simulink model "quartercar_active"  (Simulink 8.1)
settings: Solver=ode45  StartTime=0.0  StopTime=100  RelTol=1e-3
InitFcn:
  | mb=2500;
  | mw=320;
  | k1=80000;
  | k2=500000;
  | b1=320;
  | b2=15020;
  | h=1;
  | n=100;
  | g=5.01;
  | ksw=100.65;
settings Model: Creator=Sukriti Singh  LastModifiedBy=Sukriti Singh
settings DataIOCC: SignalLoggingSaveFormat=Dataset  InspectSignalLogs=on
settings OptimizationCC: ExpressionDepthLimit=128
settings DebuggingCC: FcnCallInpInsideContextMsg=EnableAllAsError
settings GRTTargetCC: CombineOutputUpdateFcns=on  GRTInterface=off

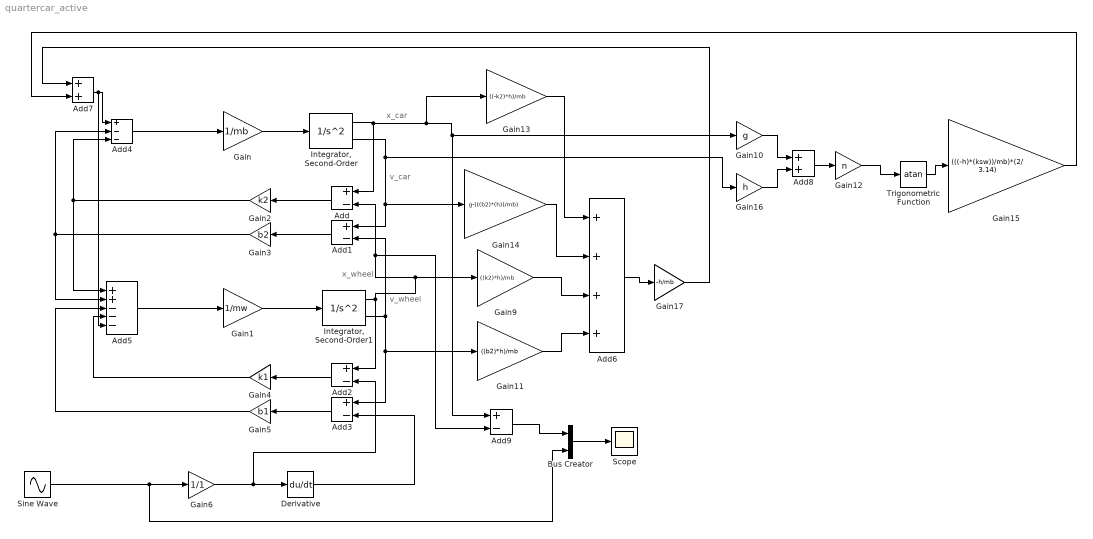
== system quartercar_active ==
  note: v_wheel
  note: x_wheel
  note: x_car
  note: v_car
  Add{,1..3,9} (5 alike) : Sum  Inputs=+-
  Add4 : Sum  Inputs=+--
  Add5 : Sum  Inputs=++---
  Add6 : Sum  Inputs=++++
  Add7 : Sum
  Add8 : Sum
  Bus Creator : BusCreator  Inputs=2
  Derivative : Derivative
  Gain : Gain  Gain=1/mb
  Gain1 : Gain  Gain=1/mw
  Gain10 : Gain  Gain=g
  Gain11 : Gain  Gain=((b2)*h)/mb
  Gain12 : Gain  Gain=n
  Gain13 : Gain  Gain=((-k2)*h)/mb
  Gain14 : Gain  Gain=g-(((b2)*(h))/mb)
  Gain15 : Gain  Gain=(((-h)*(ksw))/mb)*(2/ 3.14)
  Gain16 : Gain  Gain=h
  Gain17 : Gain  Gain=-h/mb
  Gain2 : Gain  Gain=k2
  Gain3 : Gain  Gain=b2
  Gain4 : Gain  Gain=k1
  Gain5 : Gain  Gain=b1
  Gain6 : Gain  Gain=1/1
  Gain9 : Gain  Gain=((k2)*h)/mb
  "Integrator, Second-Order" : SecondOrderIntegrator
  "Integrator, Second-Order1" : SecondOrderIntegrator
  Scope : Scope
      settings: YMax=4.5
  Sine Wave : Sin  Amplitude=0.01  Frequency=20  SampleTime=0
  Trigonometric Function : Trigonometry  Operator=atan
  wires:
  Derivative/1 -> Add3/2
  Add3/1 -> Gain5/1
  Add2/1 -> Gain4/1
  Gain1/1 -> "Integrator, Second-Order1"/1
  Add1/1 -> Gain3/1
  Add/1 -> Gain2/1
  Gain/1 -> "Integrator, Second-Order"/1
  Add4/1 -> Gain/1
  Add5/1 -> Gain1/1
  Gain2/1 -> Add5/1, Add4/3
  Gain3/1 -> Add4/2, Add5/2
  Gain4/1 -> Add5/4
  Gain5/1 -> Add5/3
  "Integrator, Second-Order"/2 -> Add1/1, Gain14/1, Gain16/1
  "Integrator, Second-Order1"/1 -> Add2/1, Add9/2, Add/2, Gain9/1
  "Integrator, Second-Order1"/2 -> Add1/2, Add3/1, Gain11/1
  Gain6/1 -> Add2/2, Derivative/1
  Sine Wave/1 -> Bus Creator/2, Gain6/1
  Gain13/1 -> Add6/1
  Gain14/1 -> Add6/2
  Gain9/1 -> Add6/3
  Gain11/1 -> Add6/4
  Add6/1 -> Gain17/1
  Gain17/1 -> Add7/1
  Gain10/1 -> Add8/1
  Add8/1 -> Gain12/1
  Gain15/1 -> Add7/2
  "Integrator, Second-Order"/1 -> Gain13/1, Add9/1, Gain10/1, Add/1
  Bus Creator/1 -> Scope/1
  Gain12/1 -> Trigonometric Function/1
  Trigonometric Function/1 -> Gain15/1
  Gain16/1 -> Add8/2
  Add7/1 -> Add5/5, Add4/1
  Add9/1 -> Bus Creator/1
